simulink model "QuadSimUnity"  (R2015b)
settings: Solver=ode4  StartTime=0.0  StopTime=inf  FixedStep=Ts  RelTol=1e-3
values from neighbouring files (symbols this model uses):
  alpha1 = 10    [QuadSimInit.m]
  alpha2 = .5    (= 0.5)    [QuadSimInit.m]
  alpha3 = 10    [QuadSimInit.m]
  alpha4 = 0.5    [QuadSimInit.m]
  alpha5 = 10    [QuadSimInit.m]
  alpha6 = 0.5    [QuadSimInit.m]
  Am = -20*diag([1, 1, 1])    [QuadSimInit.m]
  b = 3.13e-5/2    (= 1.565e-05)    [QuadSimInit.m]
  Bm = inv(I)    [QuadSimInit.m]
  d = 7.5e-7/2    (= 3.75e-07)    [QuadSimInit.m]
  D_angle = 0.2    [QuadSimInit.m]
  Delay_Act = 0.003    [QuadSimInit.m]
  g = 9.81    [QuadSimInit.m]
  I_angle = 0.1    [QuadSimInit.m]
  Inverse_Psi_nom = Psi_nom.'*inv(Psi_nom*Psi_nom.')    [QuadSimInit.m]
  Ix_0 = 7.5e-3*1    (= 0.0075)    [QuadSimInit.m]
  Iy_0 = 6.5e-3*1    (= 0.0065)    [QuadSimInit.m]
  Iz_0 = 1.3e-2*1    (= 0.013)    [QuadSimInit.m]
  Jr = 6e-5    (= 6e-05)    [QuadSimInit.m]
  K = 100    [QuadSimInit.m]
  l = 0.23    [QuadSimInit.m]
  m = 0.650*4    (= 2.6)    [QuadSimInit.m]
  P_angle = 5    [QuadSimInit.m]
  Ts = 0.001    [QuadSimInit.m]
undefined symbols (not defined in the file or in its folder): a
libraries: simulink x9, etargetslib x5, dspnetwork x5, cstblocks x1, aerolibanimutils x1
settings Model: Creator=hyoon33  LastModifiedBy=lakshma2
settings SolverCC: AutoInsertRateTranBlk=on
settings DataIOCC: SaveFormat=Array
settings DebuggingCC: UnderspecifiedInitializationDetection=Classic  MergeDetectMultiDrivingBlocksExec=none  SolverPrmCheckMsg=warning  StateNameClashWarn=warning
settings HardwareCC: ProdBitPerPointer=32  ProdLargestAtomicFloat=None  ProdIntDivRoundTo=Undefined  ProdEndianess=Unspecified  ProdWordSize=32  ProdHWDeviceType=32-bit Generic
settings GRTTargetCC: GeneratePreprocessorConditionals=Disable all
settings ConfigComp: CovModelRefEnable=Off  CovSFcnEnable=off

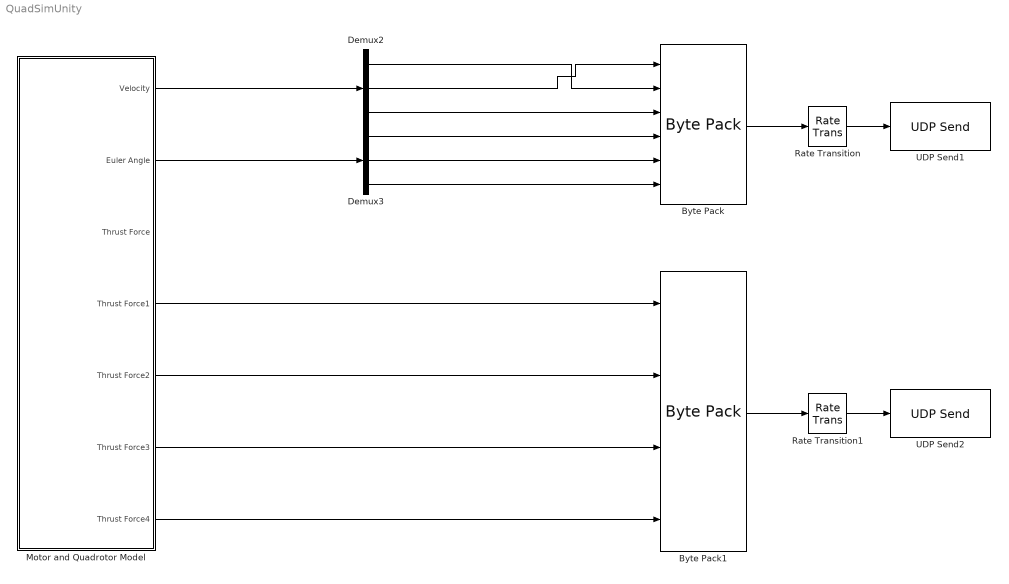
== system QuadSimUnity ==
  Byte Pack : etargetslib/Byte Pack  datatypes={'double','double','double','double','double','double'}  byteAlign=1
  Byte Pack1 : etargetslib/Byte Pack  datatypes={'double','double','double','double'}  byteAlign=1
  Demux2 : Demux  Outputs=3
  Demux3 : Demux  Outputs=3
  Motor and Quadrotor Model : Subsystem
  Rate Transition : RateTransition  OutPortSampleTime=0.016/16
  Rate Transition1 : RateTransition  OutPortSampleTime=0.016/16
  UDP Send1 : dspnetwork/UDP Send  remoteURL='127.0.0.1'  remotePort=25001  localURL='0.0.0.0'  localPortSource=Automatically determine  localPort=-1  sampletime=-1  separateLengthPort=0
  UDP Send2 : dspnetwork/UDP Send  remoteURL='127.0.0.1'  remotePort=25004  localURL='0.0.0.0'  localPortSource=Automatically determine  localPort=-1  sampletime=-1  separateLengthPort=0
  wires:
  Motor and Quadrotor Model/1(Velocity) -> Demux2/1
  Demux2/1 -> Byte Pack/2
  Demux3/2 -> Byte Pack/5
  Demux2/2 -> Byte Pack/1
  Demux3/1 -> Byte Pack/4
  Demux2/3 -> Byte Pack/3
  Demux3/3 -> Byte Pack/6
  Motor and Quadrotor Model/2(Euler Angle) -> Demux3/1
  Byte Pack/1 -> Rate Transition/1
  Rate Transition/1 -> UDP Send1/1
  Byte Pack1/1 -> Rate Transition1/1
  Rate Transition1/1 -> UDP Send2/1
  Motor and Quadrotor Model/4(Thrust Force1) -> Byte Pack1/1
  Motor and Quadrotor Model/5(Thrust Force2) -> Byte Pack1/2
  Motor and Quadrotor Model/6(Thrust Force3) -> Byte Pack1/3
  Motor and Quadrotor Model/7(Thrust Force4) -> Byte Pack1/4

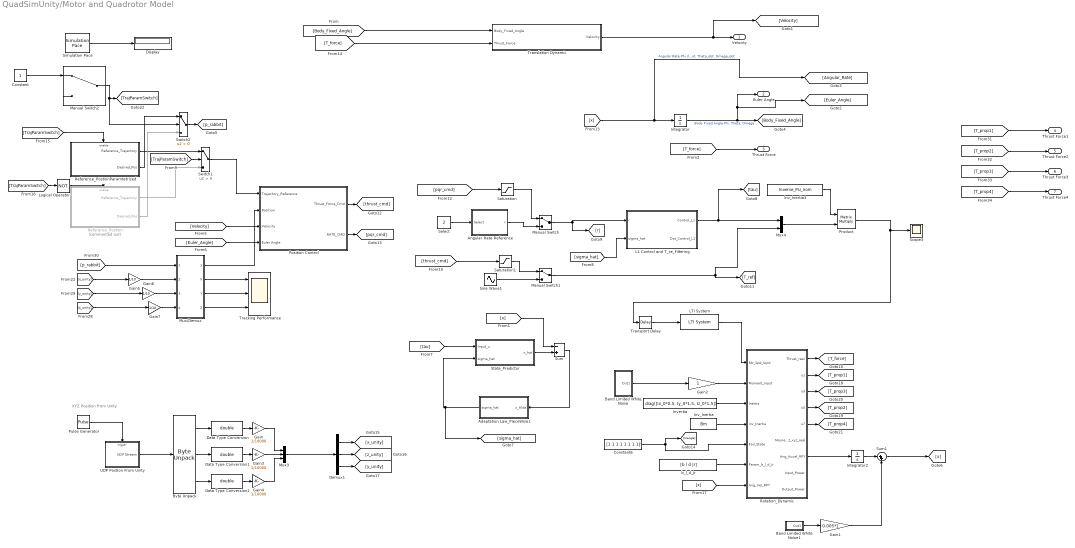
== system QuadSimUnity/Motor and Quadrotor Model ==
  note: XYZ Position from Unity
  Adaptation Law_PieceWise1 : Subsystem
  Angular Rate Reference : Subsystem
  Band Limited White Noise : Subsystem
  Band Limited White Noise1 : Subsystem
  Byte Unpack : etargetslib/Byte Unpack  dimensions={1,1,1}  datatypes={'int32','int32','int32'}  byteAlign=1
  Constant : Constant
  Constant6 : Constant  Value=[1 1 1 1 1 1 1 1]'
  Data Type Conversion : DataTypeConversion  OutDataTypeStr=double
  Data Type Conversion1 : DataTypeConversion  OutDataTypeStr=double
  Data Type Conversion2 : DataTypeConversion  OutDataTypeStr=double
  Demux1 : Demux  Outputs=3
  Display : Display
  Gain : Gain  Gain=1/10000
  Gain1 : Gain  Gain=0.005*1
  Gain2 : Gain
  Gain3 : Gain  Gain=1/10000
  Gain4 : Gain  Gain=1/10000
  Gain5 : Gain  Gain=1/10
  Gain6 : Gain  Gain=1/10
  Gain7 : Gain  Gain=1/10
  Integrator : Integrator
  Integrator2 : Integrator  InitialCondition=[0 0 0]'
  Inv_Inertia : Constant  Value=Bm  VectorParams1D=off
  Inv_Inertia3 : Constant  Value=Inverse_Psi_nom  VectorParams1D=off
  Invertia : Constant  Value=diag([Ix_0*0.5, Iy_0*1.5, Iz_0*1.5])  VectorParams1D=off
  L1 Control and T_re_Filtering : Subsystem
  LTI System : cstblocks/LTI System  sys=H_motor  IC=[]
  Logical Operator : Logic  Operator=NOT  AllPortsSameDT=off  OutDataTypeStr=boolean
  Manual Switch : ManualSwitch
  Manual Switch1 : ManualSwitch
  Manual Switch2 : ManualSwitch
  Mux/Demux : Subsystem
  Mux3 : Mux  Inputs=3
  Mux4 : Mux  Inputs=2
  Position Control : Subsystem
  Product : Product  Multiplication=Matrix(*)
  Pulse Generator : DiscretePulseGenerator  PulseType=Time based  Period=1/50  PulseWidth=50
  Reference_Postion : Subsystem  Commented=on
  Reference_PostionParamtetrized : Subsystem
  Rotation_Dynamic : MATLAB Function  TreatAsAtomicUnit=on
  Saturation : Saturate  UpperLimit=10  LowerLimit=-10
  Saturation1 : Saturate  UpperLimit=100  LowerLimit=-100
  Scope3 : Scope
  Select : Constant  Value=2
  Simulation Pace : aerolibanimutils/Simulation Pace  SimulationPace=1  SleepMode=MATLAB Thread  OutputPaceError=on  SampleTime=-1
      settings: AttributesFormatString=%<SimulationPace> sec/sec
  Sine Wave1 : Sin  Amplitude=0  Bias=m*9.81  Frequency=2  SampleTime=0
  State_Predictor : Subsystem
  Sum : Sum  Inputs=-+
  Sum1 : Sum  Inputs=|++
  Switch1 : Switch  Criteria=u2 > Threshold
  Switch2 : Switch  Criteria=u2 > Threshold
  Tracking Performance : Scope  NumInputPorts=3
  Translation Dynamic : Subsystem
  Transport Delay : TransportDelay  DelayTime=Delay_Act
  UDP Postion From Unity : Subsystem
  b_l_d_Jr : Constant  Value=[b l d Jr]
  Velocity : Outport
  Euler Angle : Outport  Port=2
  Thrust Force : Outport  Port=3
  Thrust Force1 : Outport  Port=4
  Thrust Force2 : Outport  Port=5
  Thrust Force3 : Outport  Port=6
  Thrust Force4 : Outport  Port=7
  wires:
  [Velocity] -> Position Control/3(Velocity)
  [Euler_Angle] -> Position Control/4(Euler Angle)
  [x] -> Integrator/1, [Angular_Rate]  "Angular Rate Phi dot, Theta_dot, Omega_dot"
  Integrator/1 -> Euler Angle/1, [Euler_Angle], [Body_Fixed_Angle]  "Body Fixed Angle Phi, Theta, Omega"
  [Body_Fixed_Angle] -> Translation Dynamic/1(Body_Fixed_Angle)
  b_l_d_Jr/1 -> Rotation_Dynamic/6(Param_b_l_d_Jr)
  Invertia/1 -> Rotation_Dynamic/3(Inertia)
  Inv_Inertia/1 -> Rotation_Dynamic/4(inv_Inertia)
  Rotation_Dynamic/7(Ang_Accel_RPY) -> Integrator2/1
  Manual Switch/1 -> L1 Control and T_re_Filtering/1(r), [r]
  Select/1 -> Angular Rate Reference/1(Select)
  [sigma_hat] -> L1 Control and T_re_Filtering/2(sigma_hat)
  L1 Control and T_re_Filtering/1(Control_L1) -> Mux4/1, [tau]
  Integrator2/1 -> Sum1/1
  Band Limited White Noise/1(Out1) -> Gain2/1
  Gain2/1 -> Rotation_Dynamic/2(Moment_Input)
  Transport Delay/1 -> LTI System/1
  LTI System/1 -> Rotation_Dynamic/1(Rtr_Spd_Sqrd)
  Constant6/1 -> [triangle], Rotation_Dynamic/5(Fail_State)
  State_Predictor/1(x_hat) -> Sum/2
  [x] -> Sum/1
  Sum/1 -> Adaptation Law_PieceWise1/1(x_tilda)
  Adaptation Law_PieceWise1/1(sigma_hat) -> [sigma_hat], State_Predictor/2(sigma_hat)
  Rotation_Dynamic/1(Thrust_real) -> [T_force]
  [tau] -> State_Predictor/1(input_u)
  Manual Switch1/1 -> Mux4/2, [T_ref]
  Angular Rate Reference/1(r) -> Manual Switch/2
  [pqr_cmd] -> Saturation/1
  Sine Wave1/1 -> Manual Switch1/2
  [thrust_cmd] -> Saturation1/1
  Saturation/1 -> Manual Switch/1
  Saturation1/1 -> Manual Switch1/1
  Position Control/1(Thrust_Force_Cmd) -> [thrust_cmd]
  Position Control/2(RATE_CMD) -> [pqr_cmd]
  [T_force] -> Translation Dynamic/2(Thrust_Force)
  Sum1/1 -> [x]
  Band Limited White Noise1/1(Out1) -> Gain1/1
  Gain1/1 -> Sum1/2
  Translation Dynamic/1(Velocity) -> [Velocity], Velocity/1
  Product/1 -> Transport Delay/1, Scope3/1
  [x] -> Rotation_Dynamic/7(Ang_Vel_RPY)
  Mux4/1 -> Product/2
  Inv_Inertia3/1 -> Product/1
  Byte Unpack/1 -> Data Type Conversion/1
  Byte Unpack/2 -> Data Type Conversion1/1
  Byte Unpack/3 -> Data Type Conversion2/1
  Simulation Pace/1 -> Display/1
  UDP Postion From Unity/1(UDP Stream) -> Byte Unpack/1
  Pulse Generator/1 -> UDP Postion From Unity/Trigger
  Gain/1 -> Mux3/1
  Gain3/1 -> Mux3/2
  Gain4/1 -> Mux3/3
  Data Type Conversion/1 -> Gain/1
  Data Type Conversion1/1 -> Gain3/1
  Data Type Conversion2/1 -> Gain4/1
  [p_rabbit] -> Mux/Demux/1(Rabbit)
  [x_unity] -> Gain5/1
  [y_unity] -> Gain6/1
  [z_unity] -> Gain7/1
  Mux/Demux/1(Position) -> Position Control/2(Position)
  Mux/Demux/2(X) -> Tracking Performance/1
  Mux/Demux/3(Y) -> Tracking Performance/2
  Mux/Demux/4(Z) -> Tracking Performance/3
  [T_force] -> Thrust Force/1
  Gain5/1 -> Mux/Demux/2(XUnity)
  Gain6/1 -> Mux/Demux/3(YUnity)
  Gain7/1 -> Mux/Demux/4(ZUnity)
  Mux3/1 -> Demux1/1
  Demux1/1 -> [x_unity]
  Demux1/2 -> [z_unity]
  Demux1/3 -> [y_unity]
  Rotation_Dynamic/2(u1) -> [T_prop1]
  Rotation_Dynamic/4(u5) -> [T_prop2]
  Rotation_Dynamic/3(u3) -> [T_prop3]
  Rotation_Dynamic/5(u7) -> [T_prop4]
  [T_prop1] -> Thrust Force1/1
  [T_prop2] -> Thrust Force2/1
  [T_prop3] -> Thrust Force3/1
  [T_prop4] -> Thrust Force4/1
  Switch1/1 -> Position Control/1(Trajectory_Reference)
  Reference_Postion/1(Reference_Trajectory) -> Switch1/3
  Reference_PostionParamtetrized/1(Reference_Trajectory) -> Switch1/1
  Reference_PostionParamtetrized/2(Desired_Pos) -> Switch2/1
  Reference_Postion/2(Desired_Pos) -> Switch2/3
  Switch2/1 -> [p_rabbit]
  Manual Switch2/1 -> Switch2/2, [TrajParamSwitch]
  Constant/1 -> Manual Switch2/1
  [TrajParamSwitch] -> Switch1/2
  [TrajParamSwitch] -> Reference_PostionParamtetrized/Enable
  [TrajParamSwitch] -> Logical Operator/1
  Logical Operator/1 -> Reference_Postion/Enable

== system QuadSimUnity/Motor and Quadrotor Model/Adaptation Law_PieceWise1 ==
  x_tilda : Inport
  -inv(Bm)*inv(Phi_Ts)*exp_Am_Ts : Constant  Value=inv(Bm)*inv(inv(Am)*(expm(Am*Ts)-eye(3)))*(expm(Am*Ts))
  Gain3 : Gain  Gain=-1
  Product6 : Product  Multiplication=Matrix(*)
  Rate Transition : RateTransition  OutPortSampleTime=Ts
  Rate Transition1 : RateTransition  OutPortSampleTimeOpt=Inherit  OutPortSampleTime=Ts
  Rate Transition3 : RateTransition  X0=inv(Bm)*inv(inv(Am)*(exp(Am*Ts)-eye(3)))*(exp(Am*Ts))  OutPortSampleTime=Ts
  Saturation2 : Saturate  Commented=through  UpperLimit=10000  LowerLimit=-10000
  sigma_hat : Outport
  wires:
  Saturation2/1 -> sigma_hat/1
  Rate Transition3/1 -> Product6/1
  Gain3/1 -> Rate Transition1/1
  Rate Transition1/1 -> Saturation2/1
  -inv(Bm)*inv(Phi_Ts)*exp_Am_Ts/1 -> Rate Transition3/1
  x_tilda/1 -> Rate Transition/1
  Product6/1 -> Gain3/1
  Rate Transition/1 -> Product6/2

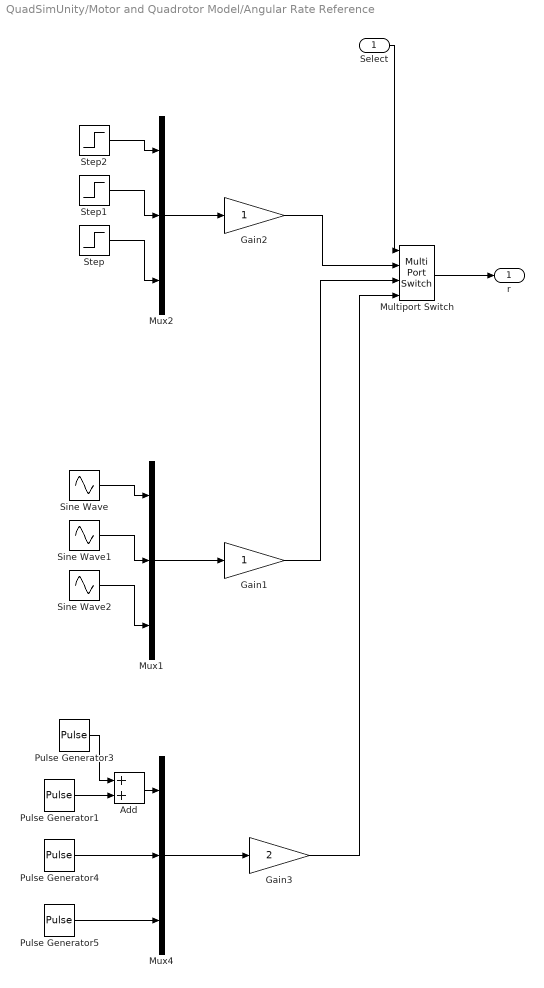
== system QuadSimUnity/Motor and Quadrotor Model/Angular Rate Reference ==
  Select : Inport
  Add : Sum
  Gain1 : Gain
  Gain2 : Gain
  Gain3 : Gain  Gain=2
  Multiport Switch : MultiPortSwitch
  Mux1 : Mux  Inputs=3
  Mux2 : Mux  Inputs=3
  Mux4 : Mux  Inputs=3
  Pulse Generator1 : DiscretePulseGenerator  PulseType=Time based  Amplitude=-1  Period=10  PhaseDelay=10
  Pulse Generator3 : DiscretePulseGenerator  PulseType=Time based  Period=10  PhaseDelay=1
  Pulse Generator4 : DiscretePulseGenerator  PulseType=Time based  Amplitude=0  Period=6  PulseWidth=40  PhaseDelay=1.5
  Pulse Generator5 : DiscretePulseGenerator  PulseType=Time based  Amplitude=0  Period=7  PulseWidth=40  PhaseDelay=2
  Sine Wave : Sin  Frequency=2  SampleTime=0
  Sine Wave1 : Sin  Frequency=2  Phase=pi  SampleTime=0
  Sine Wave2 : Sin  Amplitude=0  Frequency=2  SampleTime=0
  Step : Step  Time=3  After=0  SampleTime=0
  Step1 : Step  Time=2  SampleTime=0
  Step2 : Step  SampleTime=0
  r : Outport
  wires:
  Sine Wave/1 -> Mux1/1
  Sine Wave1/1 -> Mux1/2
  Sine Wave2/1 -> Mux1/3
  Step2/1 -> Mux2/1
  Step1/1 -> Mux2/2
  Step/1 -> Mux2/3
  Mux1/1 -> Gain1/1
  Mux2/1 -> Gain2/1
  Select/1 -> Multiport Switch/1
  Gain2/1 -> Multiport Switch/2
  Pulse Generator4/1 -> Mux4/2
  Pulse Generator5/1 -> Mux4/3
  Mux4/1 -> Gain3/1
  Gain1/1 -> Multiport Switch/3
  Gain3/1 -> Multiport Switch/4
  Multiport Switch/1 -> r/1
  Add/1 -> Mux4/1
  Pulse Generator3/1 -> Add/1
  Pulse Generator1/1 -> Add/2

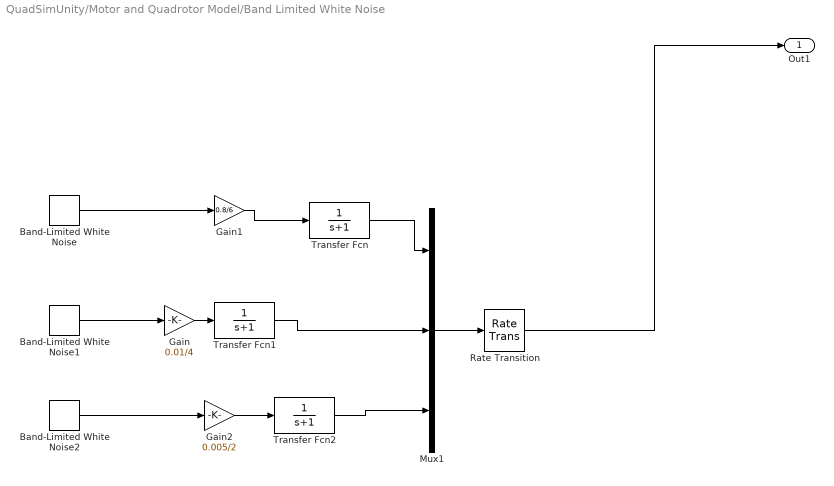
== system QuadSimUnity/Motor and Quadrotor Model/Band Limited White Noise ==
  Band-Limited White Noise : simulink/Sources/Band-Limited White Noise  Cov=[.1]  Ts=Ts  seed=[23341]
  Band-Limited White Noise1 : simulink/Sources/Band-Limited White Noise  Cov=[.1]  Ts=Ts  seed=[24451]
  Band-Limited White Noise2 : simulink/Sources/Band-Limited White Noise  Cov=[.1]  Ts=Ts  seed=[87745]
  Gain : Gain  Gain=0.01/4
  Gain1 : Gain  Gain=0.8/6
  Gain2 : Gain  Gain=0.005/2
  Mux1 : Mux  Inputs=3
  Rate Transition : RateTransition
  Transfer Fcn : TransferFcn  Denominator=[1 1]
  Transfer Fcn1 : TransferFcn  Denominator=[1 1]
  Transfer Fcn2 : TransferFcn  Denominator=[1 1]
  Out1 : Outport
  wires:
  Rate Transition/1 -> Out1/1
  Band-Limited White Noise/1 -> Gain1/1
  Band-Limited White Noise1/1 -> Gain/1
  Band-Limited White Noise2/1 -> Gain2/1
  Mux1/1 -> Rate Transition/1
  Gain/1 -> Transfer Fcn1/1
  Gain1/1 -> Transfer Fcn/1
  Gain2/1 -> Transfer Fcn2/1
  Transfer Fcn/1 -> Mux1/1
  Transfer Fcn1/1 -> Mux1/2
  Transfer Fcn2/1 -> Mux1/3

== system QuadSimUnity/Motor and Quadrotor Model/Band Limited White Noise1 ==
  Band-Limited White Noise : simulink/Sources/Band-Limited White Noise  Cov=[0.1]  Ts=0.1  seed=[23341]
  Band-Limited White Noise1 : simulink/Sources/Band-Limited White Noise  Cov=[0.1]  Ts=0.1  seed=[23241]
  Band-Limited White Noise2 : simulink/Sources/Band-Limited White Noise  Cov=[0.1]  Ts=0.1  seed=[21341]
  Mux : Mux  Inputs=3
  Rate Transition : RateTransition
  Out1 : Outport
  wires:
  Rate Transition/1 -> Out1/1
  Band-Limited White Noise1/1 -> Mux/3
  Band-Limited White Noise/1 -> Mux/1
  Mux/1 -> Rate Transition/1
  Band-Limited White Noise2/1 -> Mux/2

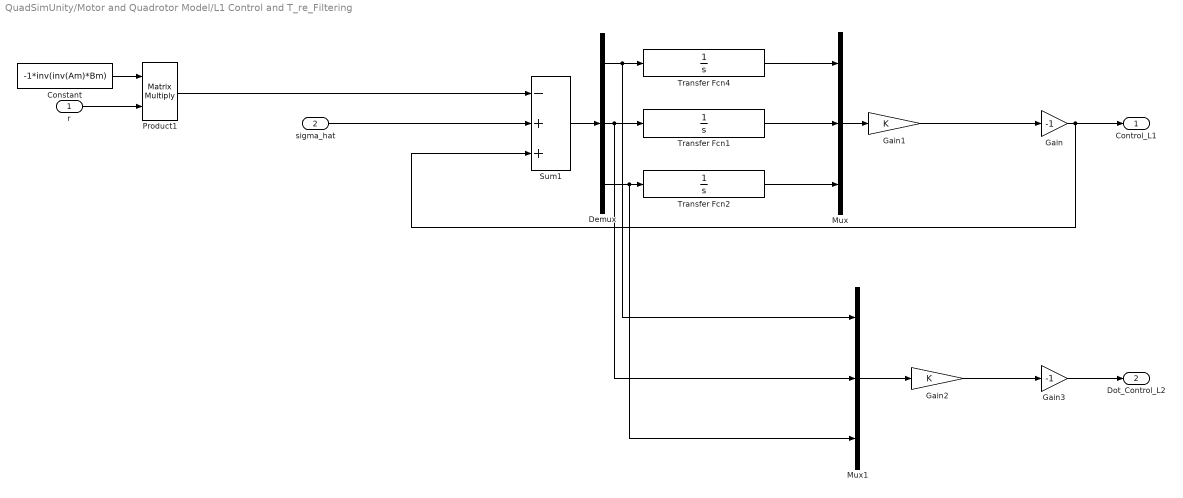
== system QuadSimUnity/Motor and Quadrotor Model/L1 Control and T_re_Filtering ==
  r : Inport
  sigma_hat : Inport  Port=2
  Constant : Constant  Value=-1*inv(inv(Am)*Bm)
  Demux : Demux  Outputs=3
  Gain : Gain  Gain=-1
  Gain1 : Gain  Gain=K
  Gain2 : Gain  Gain=K
  Gain3 : Gain  Gain=-1
  Mux : Mux  Inputs=3
  Mux1 : Mux  Inputs=3
  Product1 : Product  Multiplication=Matrix(*)
  Sum1 : Sum  Inputs=-++
  Transfer Fcn1 : TransferFcn  Denominator=[1 0]
  Transfer Fcn2 : TransferFcn  Denominator=[1 0]
  Transfer Fcn4 : TransferFcn  Denominator=[1 0]
  Control_L1 : Outport
  Dot_Control_L2 : Outport  Port=2
  wires:
  r/1 -> Product1/2
  Sum1/1 -> Demux/1
  Demux/1 -> Mux1/1, Transfer Fcn4/1
  Demux/2 -> Mux1/2, Transfer Fcn1/1
  Demux/3 -> Mux1/3, Transfer Fcn2/1
  Mux/1 -> Gain1/1
  Transfer Fcn4/1 -> Mux/1
  Transfer Fcn1/1 -> Mux/2
  Transfer Fcn2/1 -> Mux/3
  Constant/1 -> Product1/1
  sigma_hat/1 -> Sum1/2
  Gain/1 -> Sum1/3, Control_L1/1
  Product1/1 -> Sum1/1
  Gain1/1 -> Gain/1
  Mux1/1 -> Gain2/1
  Gain2/1 -> Gain3/1
  Gain3/1 -> Dot_Control_L2/1

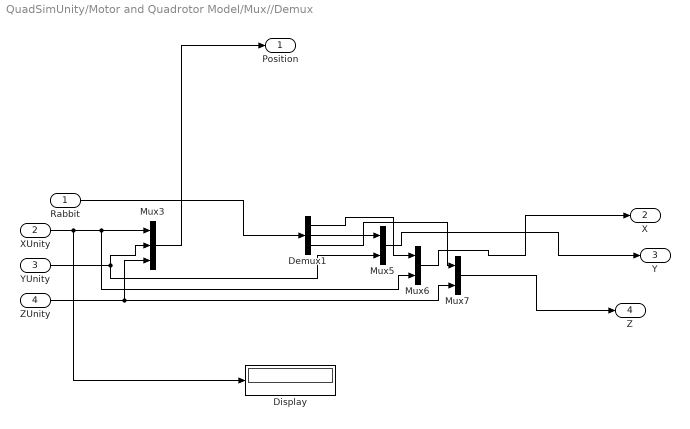
== system QuadSimUnity/Motor and Quadrotor Model/Mux//Demux ==
  Rabbit : Inport
  XUnity : Inport  Port=2
  YUnity : Inport  Port=3
  ZUnity : Inport  Port=4
  Demux1 : Demux  Outputs=3
  Display : Display
  Mux3 : Mux  Inputs=3
  Mux5 : Mux  Inputs=2
  Mux6 : Mux  Inputs=2
  Mux7 : Mux  Inputs=2
  Position : Outport
  X : Outport  Port=2
  Y : Outport  Port=3
  Z : Outport  Port=4
  wires:
  Demux1/1 -> Mux6/1
  Mux7/1 -> Z/1
  Mux6/1 -> X/1
  Demux1/2 -> Mux5/1
  Mux3/1 -> Position/1
  ZUnity/1 -> Mux3/3, Mux7/2
  YUnity/1 -> Mux3/2, Mux5/2
  XUnity/1 -> Display/1, Mux6/2, Mux3/1
  Demux1/3 -> Mux7/1
  Mux5/1 -> Y/1
  Rabbit/1 -> Demux1/1

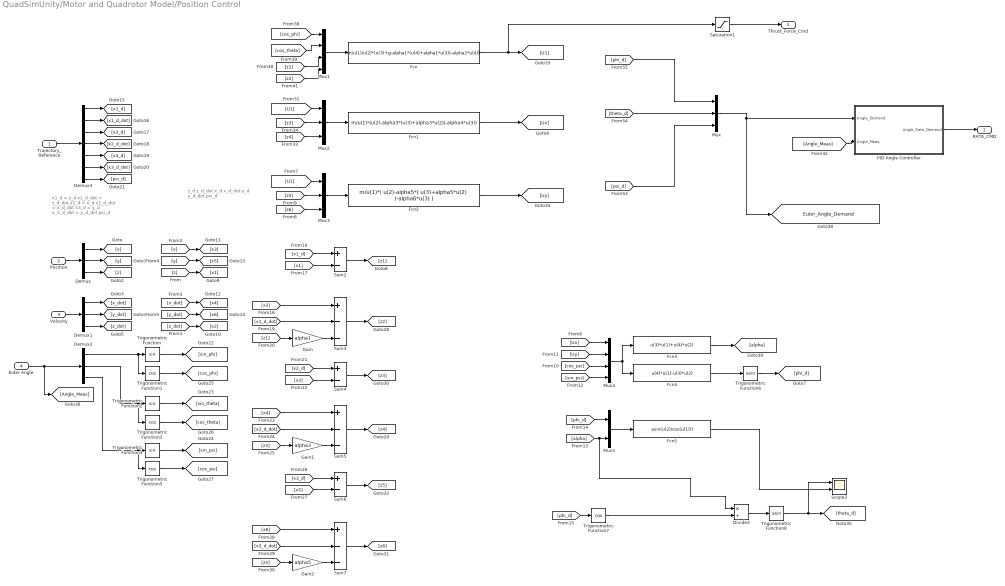
== system QuadSimUnity/Motor and Quadrotor Model/Position Control ==
  note: x1_d =  z_d
      | x1_d_dot = z_d_dot
      |
      | x2_d = x_d
      | x2_d_dot = x_d_dot
      |
      | x3_d = y_d
      | x_3_d_dot = y_d_dot
      |
      | psi_d
  note: z_d
      | z_d_dot
      |
      | x_d
      | x_d_dot
      |
      | y_d
      | y_d_dot
      |
      | psi_d
  Trajectory_Reference : Inport
  Position : Inport  Port=2
  Velocity : Inport  Port=3
  Euler Angle : Inport  Port=4
  Demux : Demux  Outputs=3
  Demux1 : Demux  Outputs=3
  Demux2 : Demux  Outputs=3
  Demux3 : Demux  Outputs=7
  Divide3 : Product  Inputs=*/
  Fcn : Fcn  Expr=m/u(1)/u(2)*(u(3)+g-alpha1*(u(4)+alpha1*u(3))-alpha2*u(4))
  Fcn1 : Fcn  Expr=m/u(1)*(u(2)-alpha3*(u(3)+alpha3*u(2))-alpha4*u(3))
  Fcn2 : Fcn  Expr=m/u(1)*( u(2)-alpha5*( u(3)+alpha5*u(2) )-alpha6*u(3) )
  Fcn3 : Fcn  Expr=u(3)*u(1)+u(4)*u(2)
  Fcn4 : Fcn  Expr=u(4)*u(1)-u(3)*u(2)
  Fcn5 : Fcn  Expr=asin(u(2)/cos(u(1)))
  Gain : Gain  Gain=alpha1
  Gain1 : Gain  Gain=alpha3
  Gain2 : Gain  Gain=alpha5
  Mux : Mux  Inputs=3
  Mux1 : Mux
  Mux2 : Mux  Inputs=3
  Mux3 : Mux  Inputs=3
  Mux4 : Mux
  Mux5 : Mux  Inputs=2
  PID Angle Controller : Subsystem
  Saturation1 : Saturate  UpperLimit=30  LowerLimit=-30
  Scope3 : Scope  NumInputPorts=2
  Sum2 : Sum  Inputs=+-
  Sum3 : Sum  Inputs=+--
  Sum4 : Sum  Inputs=+-
  Sum5 : Sum  Inputs=+--
  Sum6 : Sum  Inputs=+-
  Sum7 : Sum  Inputs=+--
  Trigonometric Function : Trigonometry
  Trigonometric Function{1,3,5,7} (4 alike) : Trigonometry  Operator=cos
  Trigonometric Function2 : Trigonometry
  Trigonometric Function4 : Trigonometry
  Trigonometric Function6 : Trigonometry  Operator=asin
  Trigonometric Function8 : Trigonometry  Operator=asin
  Thrust_Force_Cmd : Outport
  RATE_CMD : Outport  Port=2
  tag scope: Euler_Angle_Demand=global
  wires:
  Position/1 -> Demux/1
  Velocity/1 -> Demux1/1
  Euler Angle/1 -> [Angle_Meas], Demux2/1
  Demux/1 -> [x]
  Demux/2 -> [y]
  Demux/3 -> [z]
  Demux1/1 -> [x_dot]
  Demux1/2 -> [y_dot]
  Demux1/3 -> [z_dot]
  [z] -> [x1]
  [z_dot] -> [x2]
  [x] -> [x3]
  [x_dot] -> [x4]
  [y] -> [x5]
  [y_dot] -> [x6]
  Trajectory_Reference/1 -> Demux3/1
  Demux3/1 -> [x1_d]
  Demux3/2 -> [x1_d_dot]
  Demux3/3 -> [x2_d]
  Demux3/4 -> [x2_d_dot]
  Demux3/5 -> [x3_d]
  Demux3/6 -> [x3_d_dot]
  Demux3/7 -> [psi_d]
  Demux2/1 -> Trigonometric Function1/1, Trigonometric Function/1
  Trigonometric Function/1 -> [sin_phi]
  Trigonometric Function1/1 -> [cos_phi]
  Demux2/2 -> Trigonometric Function3/1, Trigonometric Function2/1
  Trigonometric Function2/1 -> [sin_theta]
  Trigonometric Function3/1 -> [cos_theta]
  Trigonometric Function4/1 -> [sin_psi]
  Trigonometric Function5/1 -> [cos_psi]
  Demux2/3 -> Trigonometric Function5/1, Trigonometric Function4/1
  [x1_d] -> Sum2/1
  [x1] -> Sum2/2
  Sum2/1 -> [z1]
  [x1_d_dot] -> Sum3/2
  [x2] -> Sum3/1
  Gain/1 -> Sum3/3
  [z1] -> Gain/1
  Sum3/1 -> [z2]
  [x2_d] -> Sum4/1
  [x3] -> Sum4/2
  Sum4/1 -> [z3]
  [x2_d_dot] -> Sum5/2
  [x4] -> Sum5/1
  Gain1/1 -> Sum5/3
  [z3] -> Gain1/1
  Sum5/1 -> [z4]
  [x3_d] -> Sum6/1
  [x5] -> Sum6/2
  Sum6/1 -> [z5]
  [x3_d_dot] -> Sum7/2
  [x6] -> Sum7/1
  Gain2/1 -> Sum7/3
  [z5] -> Gain2/1
  Sum7/1 -> [z6]
  [alpha] -> Divide3/1, Mux5/2
  Trigonometric Function7/1 -> Divide3/2
  Divide3/1 -> Trigonometric Function8/1
  Trigonometric Function8/1 -> Scope3/1, [theta_d]
  Mux1/1 -> Fcn/1
  [cos_phi] -> Mux1/1
  [cos_theta] -> Mux1/2
  [z1] -> Mux1/3
  [z2] -> Mux1/4
  Mux2/1 -> Fcn1/1
  [U1] -> Mux2/1
  [z4] -> Mux2/3
  [z3] -> Mux2/2
  Fcn1/1 -> [Ux]
  Mux3/1 -> Fcn2/1
  [U1] -> Mux3/1
  [z6] -> Mux3/3
  [z5] -> Mux3/2
  Fcn2/1 -> [Uy]
  Mux4/1 -> Fcn4/1, Fcn3/1
  [Ux] -> Mux4/1
  [cos_psi] -> Mux4/3
  [Uy] -> Mux4/2
  [sin_psi] -> Mux4/4
  Fcn4/1 -> Trigonometric Function6/1
  Trigonometric Function6/1 -> [phi_d]
  Fcn3/1 -> [alpha]
  [phi_d] -> Mux5/1
  Mux5/1 -> Fcn5/1
  Fcn5/1 -> Scope3/2
  [phi_d] -> Trigonometric Function7/1
  [phi_d] -> Mux/1
  [theta_d] -> Mux/2
  [psi_d] -> Mux/3
  Mux/1 -> PID Angle Controller/1(Angle_Demand), [Euler_Angle_Demand]
  [Angle_Meas] -> PID Angle Controller/2(Angle_Meas.)
  Saturation1/1 -> Thrust_Force_Cmd/1
  Fcn/1 -> Saturation1/1, [U1]
  PID Angle Controller/1(Angle_Rate_Demand) -> RATE_CMD/1

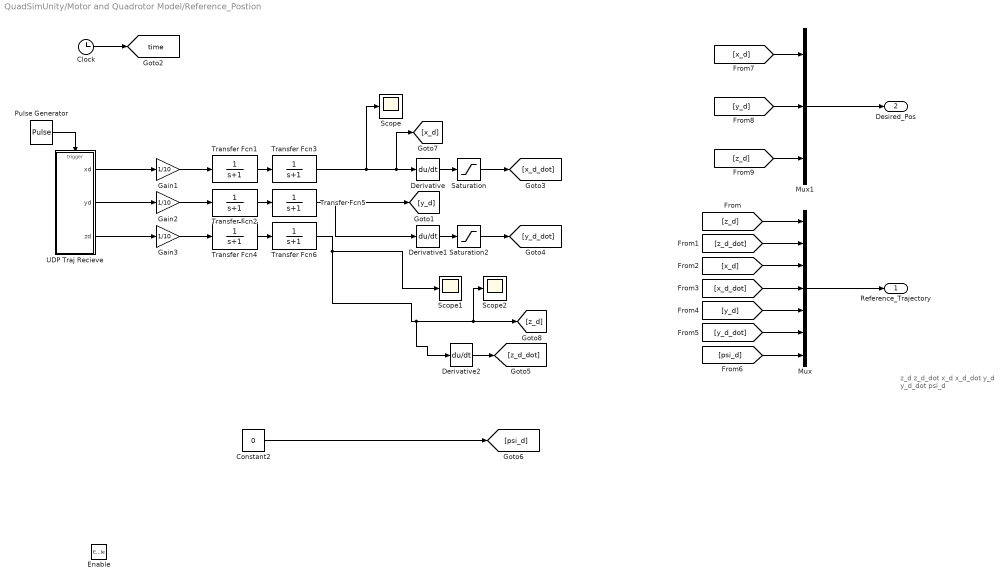
== system QuadSimUnity/Motor and Quadrotor Model/Reference_Postion ==
  note: z_d
      | z_d_dot
      |
      | x_d
      | x_d_dot
      |
      | y_d
      | y_d_dot
      |
      | psi_d
  Enable : EnablePort
  Clock : Clock
  Constant2 : Constant  Value=0
  Derivative : Derivative  CoefficientInTFapproximation=300
  Derivative1 : Derivative  CoefficientInTFapproximation=500
  Derivative2 : Derivative  CoefficientInTFapproximation=500
  Gain1 : Gain  Gain=1/10
  Gain2 : Gain  Gain=1/10
  Gain3 : Gain  Gain=1/10
  Mux : Mux  Inputs=7
  Mux1 : Mux  Inputs=3
  Pulse Generator : DiscretePulseGenerator  PulseType=Time based  Period=1/10  PulseWidth=50
  Saturation : Saturate  UpperLimit=5  LowerLimit=-5
  Saturation2 : Saturate  UpperLimit=5  LowerLimit=-5
  Scope : Scope
  Scope1 : Scope
  Scope2 : Scope
  Transfer Fcn{1..6} (6 alike) : TransferFcn  Denominator=[1 1]
  UDP Traj Recieve : Subsystem
  Reference_Trajectory : Outport
  Desired_Pos : Outport  Port=2
  tag scope: time=global
  wires:
  Constant2/1 -> [psi_d]
  Mux/1 -> Reference_Trajectory/1
  [z_d] -> Mux/1
  [z_d_dot] -> Mux/2
  [x_d] -> Mux/3
  [x_d_dot] -> Mux/4
  [y_d] -> Mux/5
  [y_d_dot] -> Mux/6
  [psi_d] -> Mux/7
  Derivative/1 -> Saturation/1
  Derivative1/1 -> Saturation2/1
  [x_d] -> Mux1/1
  [y_d] -> Mux1/2
  [z_d] -> Mux1/3
  Mux1/1 -> Desired_Pos/1
  Clock/1 -> [time]
  Transfer Fcn4/1 -> Transfer Fcn6/1
  Transfer Fcn2/1 -> Transfer Fcn5/1
  Transfer Fcn1/1 -> Transfer Fcn3/1
  Pulse Generator/1 -> UDP Traj Recieve/Trigger
  Saturation/1 -> [x_d_dot]
  UDP Traj Recieve/1(xd) -> Gain1/1
  UDP Traj Recieve/2(yd) -> Gain2/1
  UDP Traj Recieve/3(zd) -> Gain3/1
  Derivative2/1 -> [z_d_dot]
  Gain1/1 -> Transfer Fcn1/1
  Gain2/1 -> Transfer Fcn2/1
  Gain3/1 -> Transfer Fcn4/1
  Saturation2/1 -> [y_d_dot]
  Transfer Fcn3/1 -> Scope/1, [x_d], Derivative/1
  Transfer Fcn5/1 -> [y_d], Derivative1/1
  Transfer Fcn6/1 -> Derivative2/1, Scope2/1, [z_d], Scope1/1

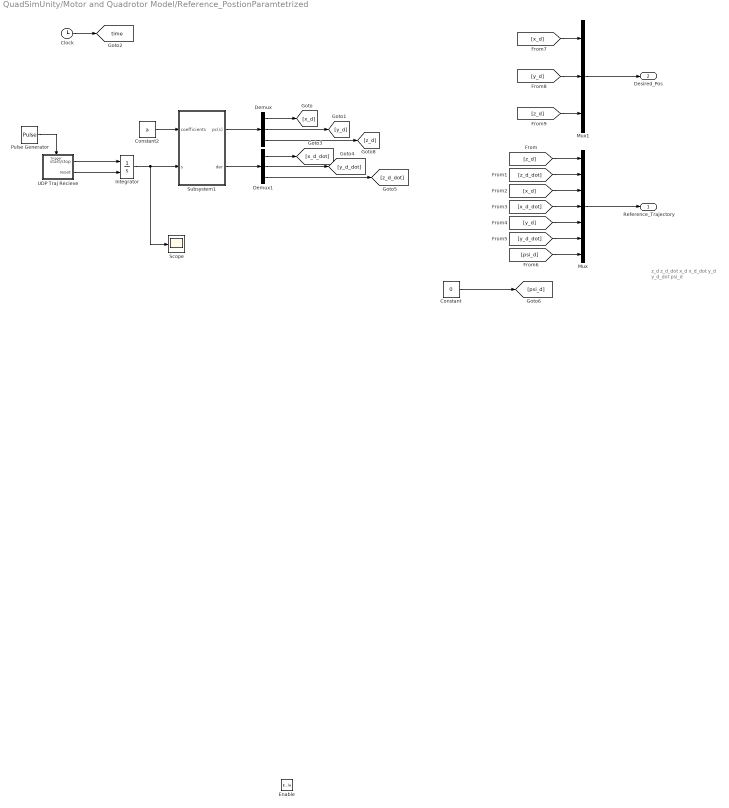
== system QuadSimUnity/Motor and Quadrotor Model/Reference_PostionParamtetrized ==
  note: z_d
      | z_d_dot
      |
      | x_d
      | x_d_dot
      |
      | y_d
      | y_d_dot
      |
      | psi_d
  Enable : EnablePort
  Clock : Clock
  Constant : Constant  Value=0
  Constant2 : Constant  Value=a
  Demux : Demux  Outputs=3
  Demux1 : Demux  Outputs=3
  Integrator : Integrator  ExternalReset=either
  Mux : Mux  Inputs=7
  Mux1 : Mux  Inputs=3
  Pulse Generator : DiscretePulseGenerator  PulseType=Time based  Period=1/50  PulseWidth=50
  Scope : Scope
  Subsystem1 : Subsystem
  UDP Traj Recieve : Subsystem
  Reference_Trajectory : Outport
  Desired_Pos : Outport  Port=2
  tag scope: time=global
  wires:
  Mux/1 -> Reference_Trajectory/1
  [z_d] -> Mux/1
  [z_d_dot] -> Mux/2
  [x_d] -> Mux/3
  [x_d_dot] -> Mux/4
  [y_d] -> Mux/5
  [y_d_dot] -> Mux/6
  [psi_d] -> Mux/7
  [x_d] -> Mux1/1
  [y_d] -> Mux1/2
  [z_d] -> Mux1/3
  Mux1/1 -> Desired_Pos/1
  Clock/1 -> [time]
  Pulse Generator/1 -> UDP Traj Recieve/Trigger
  Demux1/1 -> [x_d_dot]
  UDP Traj Recieve/1(start/stop) -> Integrator/1
  Demux1/2 -> [y_d_dot]
  Constant/1 -> [psi_d]
  Subsystem1/1(pc(s)) -> Demux/1
  Demux/1 -> [x_d]
  Demux/2 -> [y_d]
  Demux/3 -> [z_d]
  Subsystem1/2(der) -> Demux1/1
  Demux1/3 -> [z_d_dot]
  Constant2/1 -> Subsystem1/1(coefficients)
  UDP Traj Recieve/2(reset) -> Integrator/2
  Integrator/1 -> Scope/1, Subsystem1/2(s)

== system QuadSimUnity/Motor and Quadrotor Model/State_Predictor ==
  input_u : Inport
  sigma_hat : Inport  Port=2
  Am : Constant  Value=Am
  Constant4 : Constant  Value=Bm
  Integrator : Integrator
  Product : Product  Multiplication=Matrix(*)  RndMeth=Zero
  Product6 : Product  Multiplication=Matrix(*)
  Sum : Sum
  Sum1 : Sum
  x_hat : Outport
  wires:
  Product6/1 -> Sum/1
  Product/1 -> Sum/2
  Sum1/1 -> Product6/2
  Constant4/1 -> Product6/1
  Sum/1 -> Integrator/1
  input_u/1 -> Sum1/1
  Am/1 -> Product/1
  Integrator/1 -> x_hat/1, Product/2
  sigma_hat/1 -> Sum1/2

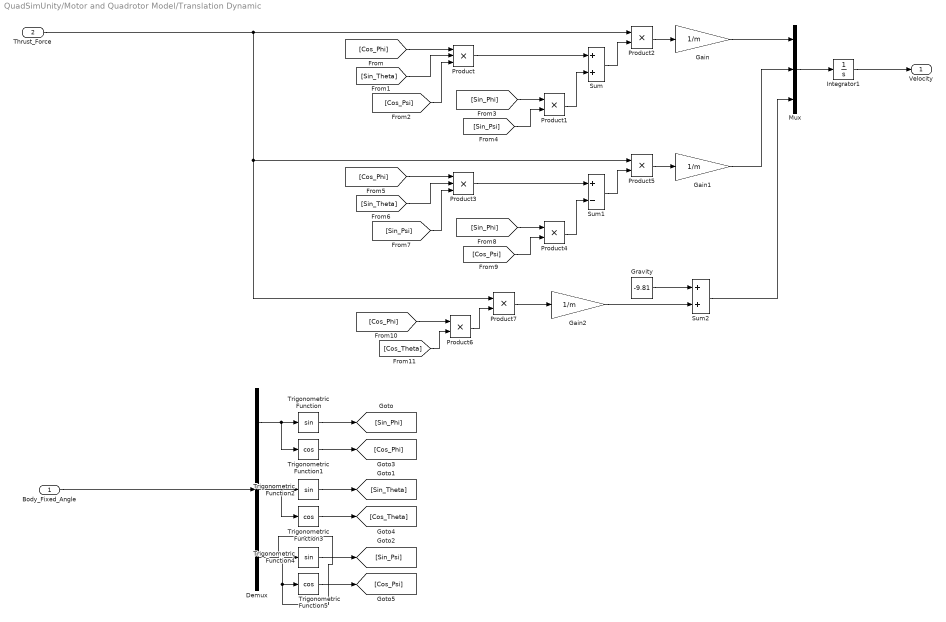
== system QuadSimUnity/Motor and Quadrotor Model/Translation Dynamic ==
  Body_Fixed_Angle : Inport
  Thrust_Force : Inport  Port=2
  Demux : Demux  Outputs=3
  Gain : Gain  Gain=1/m
  Gain1 : Gain  Gain=1/m
  Gain2 : Gain  Gain=1/m
  Gravity : Constant  Value=-9.81
  Integrator1 : Integrator  InitialCondition=[0 0 0]
  Mux : Mux  Inputs=3
  Product : Product  Inputs=3
  Product{1..2,4..7} (6 alike) : Product
  Product3 : Product  Inputs=3
  Sum : Sum
  Sum1 : Sum  Inputs=+-
  Sum2 : Sum
  Trigonometric Function : Trigonometry
  Trigonometric Function1 : Trigonometry  Operator=cos
  Trigonometric Function2 : Trigonometry
  Trigonometric Function3 : Trigonometry  Operator=cos
  Trigonometric Function4 : Trigonometry
  Trigonometric Function5 : Trigonometry  Operator=cos
  Velocity : Outport
  wires:
  Body_Fixed_Angle/1 -> Demux/1
  Demux/1 -> Trigonometric Function/1, Trigonometric Function1/1
  Trigonometric Function/1 -> [Sin_Phi]
  Trigonometric Function1/1 -> [Cos_Phi]
  Demux/2 -> Trigonometric Function3/1, Trigonometric Function2/1
  Trigonometric Function2/1 -> [Sin_Theta]
  Trigonometric Function3/1 -> [Cos_Theta]
  Trigonometric Function4/1 -> [Sin_Psi]
  Trigonometric Function5/1 -> [Cos_Psi]
  Demux/3 -> Trigonometric Function4/1, Trigonometric Function5/1
  [Cos_Phi] -> Product/1
  [Sin_Theta] -> Product/2
  [Cos_Psi] -> Product/3
  Product/1 -> Sum/1
  [Sin_Phi] -> Product1/1
  [Sin_Psi] -> Product1/2
  Product1/1 -> Sum/2
  Sum/1 -> Product2/2
  Product2/1 -> Gain/1
  [Cos_Phi] -> Product3/1
  [Sin_Theta] -> Product3/2
  [Sin_Psi] -> Product3/3
  Product3/1 -> Sum1/1
  [Sin_Phi] -> Product4/1
  [Cos_Psi] -> Product4/2
  Product4/1 -> Sum1/2
  Sum1/1 -> Product5/2
  Thrust_Force/1 -> Product7/1, Product5/1, Product2/1
  Product5/1 -> Gain1/1
  Gain1/1 -> Mux/2
  [Cos_Phi] -> Product6/1
  [Cos_Theta] -> Product6/2
  Product7/1 -> Gain2/1
  Gain2/1 -> Sum2/2
  Gravity/1 -> Sum2/1
  Product6/1 -> Product7/2
  Gain/1 -> Mux/1
  Sum2/1 -> Mux/3
  Mux/1 -> Integrator1/1
  Integrator1/1 -> Velocity/1

== system QuadSimUnity/Motor and Quadrotor Model/UDP Postion From Unity ==
  Trigger : TriggerPort  PortDimensions=1
  UDP Receive : dspnetwork/UDP Receive  localURL='0.0.0.0'  localPort=3000  remoteURL='127.0.0.1'  remotePort=-1  recvBufferSize=24  dims=12  signalDatatype=uint8  isVarSize=off  showBlockingTime=on  blockingTime=0  sampletime=-1  blockPlatform=HOST
  UDP Stream : Outport
  wires:
  UDP Receive/1 -> UDP Stream/1

== system QuadSimUnity/Motor and Quadrotor Model/Position Control/PID Angle Controller ==
  Angle_Demand : Inport
  Angle_Meas. : Inport  Port=2
  Demux : Demux  Outputs=3
  Demux1 : Demux  Outputs=3
  Mux : Mux  Inputs=3
  PID Controller (2DOF) : simulink/Continuous/PID Controller (2DOF)  Controller=PID  TimeDomain=Continuous-time  SampleTime=-1  IntegratorMethod=Forward Euler  FilterMethod=Forward Euler  Form=Parallel  UseFilter=on  ControllerParametersSource=internal  P=P_angle  I=I_angle  D=D_angle  N=100  b=1  c=1  InitialConditionSource=internal  InitialConditionForIntegrator=0  InitialConditionForFilter=0  ExternalReset=none  LimitOutput=off  UpperSaturationLimit=inf  LowerSaturationLimit=-inf  LinearizeAsGain=on  AntiWindupMode=none  Kb=1  TrackingMode=off  Kt=1  PParamMin=[]  PParamMax=[]  IParamMin=[]  IParamMax=[]  DParamMin=[]  DParamMax=[]  NParamMin=[]  NParamMax=[]  bParamMin=[]  bParamMax=[]  cParamMin=[]  cParamMax=[]  KbParamMin=[]  KbParamMax=[]  KtParamMin=[]  KtParamMax=[]  POutMin=[]  POutMax=[]  IOutMin=[]  IOutMax=[]  DOutMin=[]  DOutMax=[]  NOutMin=[]  NOutMax=[]  bOutMin=[]  bOutMax=[]  cOutMin=[]  cOutMax=[]  KbOutMin=[]  KbOutMax=[]  KtOutMin=[]  KtOutMax=[]  IntegratorOutMin=[]  IntegratorOutMax=[]  FilterOutMin=[]  FilterOutMax=[]  SumOutMin=[]  SumOutMax=[]  Sum1OutMin=[]  Sum1OutMax=[]  Sum2OutMin=[]  Sum2OutMax=[]  Sum3OutMin=[]  Sum3OutMax=[]  SumI1OutMin=[]  SumI1OutMax=[]  SumI2OutMin=[]  SumI2OutMax=[]  SumI3OutMin=[]  SumI3OutMax=[]  SumDOutMin=[]  SumDOutMax=[]  SaturationOutMin=[]  SaturationOutMax=[]  IntegratorContinuousStateAttributes=''  IntegratorStateMustResolveToSignalObject=off  IntegratorRTWStateStorageClass=Auto  FilterContinuousStateAttributes=''  FilterStateMustResolveToSignalObject=off  FilterRTWStateStorageClass=Auto  DifferentiatorICPrevScaledInput=0  DifferentiatorOutMin=[]  DifferentiatorOutMax=[]
  PID Controller (2DOF)1 : simulink/Continuous/PID Controller (2DOF)  Controller=PID  TimeDomain=Continuous-time  SampleTime=-1  IntegratorMethod=Forward Euler  FilterMethod=Forward Euler  Form=Parallel  UseFilter=on  ControllerParametersSource=internal  P=P_angle  I=I_angle  D=D_angle  N=100  b=1  c=1  InitialConditionSource=internal  InitialConditionForIntegrator=0  InitialConditionForFilter=0  ExternalReset=none  LimitOutput=off  UpperSaturationLimit=inf  LowerSaturationLimit=-inf  LinearizeAsGain=on  AntiWindupMode=none  Kb=1  TrackingMode=off  Kt=1  PParamMin=[]  PParamMax=[]  IParamMin=[]  IParamMax=[]  DParamMin=[]  DParamMax=[]  NParamMin=[]  NParamMax=[]  bParamMin=[]  bParamMax=[]  cParamMin=[]  cParamMax=[]  KbParamMin=[]  KbParamMax=[]  KtParamMin=[]  KtParamMax=[]  POutMin=[]  POutMax=[]  IOutMin=[]  IOutMax=[]  DOutMin=[]  DOutMax=[]  NOutMin=[]  NOutMax=[]  bOutMin=[]  bOutMax=[]  cOutMin=[]  cOutMax=[]  KbOutMin=[]  KbOutMax=[]  KtOutMin=[]  KtOutMax=[]  IntegratorOutMin=[]  IntegratorOutMax=[]  FilterOutMin=[]  FilterOutMax=[]  SumOutMin=[]  SumOutMax=[]  Sum1OutMin=[]  Sum1OutMax=[]  Sum2OutMin=[]  Sum2OutMax=[]  Sum3OutMin=[]  Sum3OutMax=[]  SumI1OutMin=[]  SumI1OutMax=[]  SumI2OutMin=[]  SumI2OutMax=[]  SumI3OutMin=[]  SumI3OutMax=[]  SumDOutMin=[]  SumDOutMax=[]  SaturationOutMin=[]  SaturationOutMax=[]  IntegratorContinuousStateAttributes=''  IntegratorStateMustResolveToSignalObject=off  IntegratorRTWStateStorageClass=Auto  FilterContinuousStateAttributes=''  FilterStateMustResolveToSignalObject=off  FilterRTWStateStorageClass=Auto  DifferentiatorICPrevScaledInput=0  DifferentiatorOutMin=[]  DifferentiatorOutMax=[]
  PID Controller (2DOF)2 : simulink/Continuous/PID Controller (2DOF)  Controller=PID  TimeDomain=Continuous-time  SampleTime=-1  IntegratorMethod=Forward Euler  FilterMethod=Forward Euler  Form=Parallel  UseFilter=on  ControllerParametersSource=internal  P=P_angle  I=I_angle  D=D_angle  N=100  b=1  c=1  InitialConditionSource=internal  InitialConditionForIntegrator=0  InitialConditionForFilter=0  ExternalReset=none  LimitOutput=off  UpperSaturationLimit=inf  LowerSaturationLimit=-inf  LinearizeAsGain=on  AntiWindupMode=none  Kb=1  TrackingMode=off  Kt=1  PParamMin=[]  PParamMax=[]  IParamMin=[]  IParamMax=[]  DParamMin=[]  DParamMax=[]  NParamMin=[]  NParamMax=[]  bParamMin=[]  bParamMax=[]  cParamMin=[]  cParamMax=[]  KbParamMin=[]  KbParamMax=[]  KtParamMin=[]  KtParamMax=[]  POutMin=[]  POutMax=[]  IOutMin=[]  IOutMax=[]  DOutMin=[]  DOutMax=[]  NOutMin=[]  NOutMax=[]  bOutMin=[]  bOutMax=[]  cOutMin=[]  cOutMax=[]  KbOutMin=[]  KbOutMax=[]  KtOutMin=[]  KtOutMax=[]  IntegratorOutMin=[]  IntegratorOutMax=[]  FilterOutMin=[]  FilterOutMax=[]  SumOutMin=[]  SumOutMax=[]  Sum1OutMin=[]  Sum1OutMax=[]  Sum2OutMin=[]  Sum2OutMax=[]  Sum3OutMin=[]  Sum3OutMax=[]  SumI1OutMin=[]  SumI1OutMax=[]  SumI2OutMin=[]  SumI2OutMax=[]  SumI3OutMin=[]  SumI3OutMax=[]  SumDOutMin=[]  SumDOutMax=[]  SaturationOutMin=[]  SaturationOutMax=[]  IntegratorContinuousStateAttributes=''  IntegratorStateMustResolveToSignalObject=off  IntegratorRTWStateStorageClass=Auto  FilterContinuousStateAttributes=''  FilterStateMustResolveToSignalObject=off  FilterRTWStateStorageClass=Auto  DifferentiatorICPrevScaledInput=0  DifferentiatorOutMin=[]  DifferentiatorOutMax=[]
  Scope : Scope  NumInputPorts=2
  Sum : Sum  Inputs=|+-
  Angle_Rate_Demand : Outport
  wires:
  Demux1/2 -> PID Controller (2DOF)1/2
  Demux/2 -> PID Controller (2DOF)1/1
  Angle_Meas./1 -> Demux1/1, Sum/2
  Demux1/1 -> PID Controller (2DOF)/2
  Demux/1 -> PID Controller (2DOF)/1
  Demux1/3 -> PID Controller (2DOF)2/2
  Angle_Demand/1 -> Scope/1, Sum/1, Demux/1
  Demux/3 -> PID Controller (2DOF)2/1
  PID Controller (2DOF)/1 -> Mux/1
  PID Controller (2DOF)1/1 -> Mux/2
  PID Controller (2DOF)2/1 -> Mux/3
  Mux/1 -> Angle_Rate_Demand/1
  Sum/1 -> Scope/2

== system QuadSimUnity/Motor and Quadrotor Model/Reference_Postion/UDP Traj Recieve ==
  Trigger : TriggerPort  PortDimensions=1
  Byte Unpack1 : etargetslib/Byte Unpack  dimensions={1,1,1}  datatypes={'double','double','double'}  byteAlign=1
  UDP Receive : dspnetwork/UDP Receive  localURL='0.0.0.0'  localPort=25002  remoteURL='127.0.0.1'  remotePort=-1  recvBufferSize=24  dims=24  signalDatatype=uint8  isVarSize=off  showBlockingTime=on  blockingTime=0  sampletime=-1  blockPlatform=HOST
  xd : Outport
  yd : Outport  Port=2
  zd : Outport  Port=3
  wires:
  UDP Receive/1 -> Byte Unpack1/1
  Byte Unpack1/1 -> xd/1
  Byte Unpack1/2 -> yd/1
  Byte Unpack1/3 -> zd/1

== system QuadSimUnity/Motor and Quadrotor Model/Reference_PostionParamtetrized/Subsystem1 ==
  coefficients : Inport
  s : Inport  Port=2
  polynomial : Product  Multiplication=Matrix(*)  SaturateOnIntegerOverflow=on  OutDataTypeStr=Inherit: Same as first input
  polynomial1 : Product  Multiplication=Matrix(*)  SaturateOnIntegerOverflow=on  OutDataTypeStr=Inherit: Same as first input
  tau vector : Subsystem
  tau vector1 : Subsystem
  pc(s) : Outport
  der : Outport  Port=2
  wires:
  polynomial/1 -> pc(s)/1
  tau vector/1(tau_vector) -> polynomial/2
  tau vector1/1(tau_vector) -> polynomial1/2
  s/1 -> tau vector1/1(tau), tau vector/1(tau)
  coefficients/1 -> polynomial1/1, polynomial/1
  polynomial1/1 -> der/1

== system QuadSimUnity/Motor and Quadrotor Model/Reference_PostionParamtetrized/UDP Traj Recieve ==
  Trigger : TriggerPort  PortDimensions=1
  Byte Unpack1 : etargetslib/Byte Unpack  dimensions={1,1}  datatypes={'int8','int8'}  byteAlign=1
  Data Type Conversion : DataTypeConversion  OutDataTypeStr=double
  Data Type Conversion1 : DataTypeConversion  OutDataTypeStr=double
  UDP Receive : dspnetwork/UDP Receive  localURL='0.0.0.0'  localPort=25002  remoteURL='127.0.0.1'  remotePort=-1  recvBufferSize=2  dims=2  signalDatatype=uint8  isVarSize=off  showBlockingTime=on  blockingTime=0  sampletime=-1  blockPlatform=HOST
  start/stop : Outport
  reset : Outport  Port=2
  wires:
  UDP Receive/1 -> Byte Unpack1/1
  Byte Unpack1/1 -> Data Type Conversion/1
  Byte Unpack1/2 -> Data Type Conversion1/1
  Data Type Conversion/1 -> start/stop/1
  Data Type Conversion1/1 -> reset/1

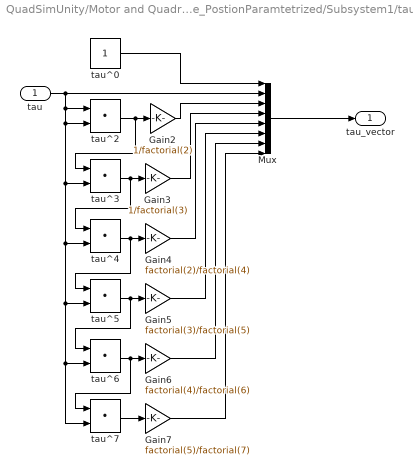
== system QuadSimUnity/Motor and Quadrotor Model/Reference_PostionParamtetrized/Subsystem1/tau vector ==
  tau : Inport
  Gain2 : Gain  Gain=1/factorial(2)  SaturateOnIntegerOverflow=on  OutDataTypeStr=Inherit: Same as input  ParamDataTypeStr=Inherit: Same as input
  Gain3 : Gain  Gain=1/factorial(3)  SaturateOnIntegerOverflow=on  OutDataTypeStr=Inherit: Same as input  ParamDataTypeStr=Inherit: Same as input
  Gain4 : Gain  Gain=factorial(2)/factorial(4)  SaturateOnIntegerOverflow=on  OutDataTypeStr=Inherit: Same as input  ParamDataTypeStr=Inherit: Same as input
  Gain5 : Gain  Gain=factorial(3)/factorial(5)  SaturateOnIntegerOverflow=on  OutDataTypeStr=Inherit: Same as input  ParamDataTypeStr=Inherit: Same as input
  Gain6 : Gain  Gain=factorial(4)/factorial(6)  SaturateOnIntegerOverflow=on  OutDataTypeStr=Inherit: Same as input  ParamDataTypeStr=Inherit: Same as input
  Gain7 : Gain  Gain=factorial(5)/factorial(7)  SaturateOnIntegerOverflow=on  OutDataTypeStr=Inherit: Same as input  ParamDataTypeStr=Inherit: Same as input
  Mux : Mux  Inputs=8
  tau^0 : Constant
  tau^{2..7} (6 alike) : DotProduct  InputSameDT=on  OutDataTypeStr=Inherit: Inherit via internal rule
  tau_vector : Outport
  wires:
  tau^6/1 -> tau^7/1, Gain6/1
  tau^7/1 -> Gain7/1
  Gain7/1 -> Mux/8
  Gain6/1 -> Mux/7
  Gain4/1 -> Mux/5
  Gain5/1 -> Mux/6
  tau^5/1 -> tau^6/1, Gain5/1
  Gain2/1 -> Mux/3
  Gain3/1 -> Mux/4
  tau^4/1 -> tau^5/1, Gain4/1
  tau^2/1 -> Gain2/1, tau^3/1
  tau^0/1 -> Mux/1
  tau^3/1 -> Gain3/1, tau^4/1
  tau/1 -> tau^7/2, tau^6/2, tau^5/2, tau^4/2, tau^3/2, tau^2/2, tau^2/1, Mux/2
  Mux/1 -> tau_vector/1

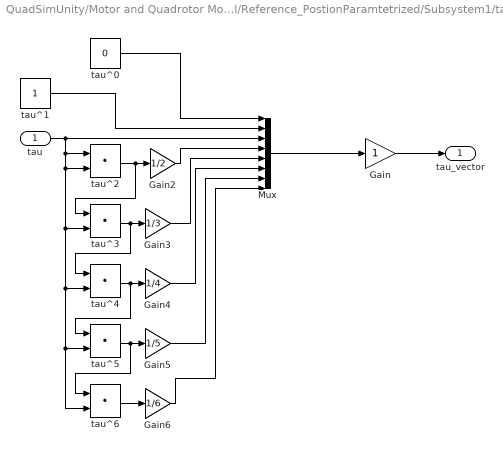
== system QuadSimUnity/Motor and Quadrotor Model/Reference_PostionParamtetrized/Subsystem1/tau vector1 ==
  tau : Inport
  Gain : Gain
  Gain2 : Gain  Gain=1/2  SaturateOnIntegerOverflow=on  OutDataTypeStr=Inherit: Same as input  ParamDataTypeStr=Inherit: Same as input
  Gain3 : Gain  Gain=1/3  SaturateOnIntegerOverflow=on  OutDataTypeStr=Inherit: Same as input  ParamDataTypeStr=Inherit: Same as input
  Gain4 : Gain  Gain=1/4  SaturateOnIntegerOverflow=on  OutDataTypeStr=Inherit: Same as input  ParamDataTypeStr=Inherit: Same as input
  Gain5 : Gain  Gain=1/5  SaturateOnIntegerOverflow=on  OutDataTypeStr=Inherit: Same as input  ParamDataTypeStr=Inherit: Same as input
  Gain6 : Gain  Gain=1/6  SaturateOnIntegerOverflow=on  OutDataTypeStr=Inherit: Same as input  ParamDataTypeStr=Inherit: Same as input
  Mux : Mux  Inputs=8
  tau^0 : Constant  Value=0
  tau^1 : Constant
  tau^{2..6} (5 alike) : DotProduct  InputSameDT=on  OutDataTypeStr=Inherit: Inherit via internal rule
  tau_vector : Outport
  wires:
  Mux/1 -> Gain/1
  tau^0/1 -> Mux/1
  tau/1 -> Mux/3, tau^2/1, tau^2/2, tau^3/2, tau^4/2, tau^5/2, tau^6/2
  tau^3/1 -> tau^4/1, Gain3/1
  tau^2/1 -> tau^3/1, Gain2/1
  tau^4/1 -> Gain4/1, tau^5/1
  Gain3/1 -> Mux/5
  Gain2/1 -> Mux/4
  tau^5/1 -> Gain5/1, tau^6/1
  Gain5/1 -> Mux/7
  Gain4/1 -> Mux/6
  Gain6/1 -> Mux/8
  tau^6/1 -> Gain6/1
  tau^1/1 -> Mux/2
  Gain/1 -> tau_vector/1

== matlab function QuadSimUnity/Motor and Quadrotor Model/Rotation_Dynamic ==
  data: Thrust_real output; u1 output; u3 output; u5 output; u7 output; Moment_xyz_real output; Rtr_Spd_Sqrd input; Moment_Input input; Inertia input; inv_Inertia input; Fail_State input; Param_b_l_d_Jr input; Ang_Vel_RPY input; Ang_Accel_RPY output; Input_Power output; Output_Power output
function [Thrust_real,u1,u3,u5,u7, Moment_xyz_real, Ang_Accel_RPY, Input_Power, Output_Power]  = fcn(Rtr_Spd_Sqrd, Moment_Input, Inertia, inv_Inertia, Fail_State, Param_b_l_d_Jr, Ang_Vel_RPY)
                
b = Param_b_l_d_Jr(1);
l = Param_b_l_d_Jr(2);
d = Param_b_l_d_Jr(3);
Jr = Param_b_l_d_Jr(4);

u1 = Rtr_Spd_Sqrd(1); u2 = Rtr_Spd_Sqrd(2); u3 = Rtr_Spd_Sqrd(3); u4 = Rtr_Spd_Sqrd(4); 
u5 = Rtr_Spd_Sqrd(5); u6 = Rtr_Spd_Sqrd(6); u7 = Rtr_Spd_Sqrd(7); u8 = Rtr_Spd_Sqrd(8); 

Input_Power = sum(Rtr_Spd_Sqrd.*Rtr_Spd_Sqrd);

Output_Power = sum((diag(Fail_State)*Rtr_Spd_Sqrd).*(diag(Fail_State)*Rtr_Spd_Sqrd));

Phi_M = ...
... 
[       0,       0, b*l*u3, b*l*u4,      0,      0, -b*l*u7, -b*l*u8; ...
  -b*l*u1, -b*l*u2,      0,      0, b*l*u5, b*l*u6,       0,       0; ...
    -d*u1,    d*u2,   d*u3,  -d*u4,  -d*u5,   d*u6,    d*u7,   -d*u8];

Phi_T = ...
... 
[ b*u1, b*u2, b*u3, b*u4, b*u5, b*u6, b*u7, b*u8];

Thrust_real = Phi_T * Fail_State;


Rtr_Spd_sum = [sqrt(abs(Rtr_Spd_Sqrd(1)))*sign(Rtr_Spd_Sqrd(1)), ...
             -sqrt(abs(Rtr_Spd_Sqrd(2)))*sign(Rtr_Spd_Sqrd(2)), ...
             sqrt(abs(Rtr_Spd_Sqrd(3)))*sign(Rtr_Spd_Sqrd(3)), ...
             -sqrt(abs(Rtr_Spd_Sqrd(4)))*sign(Rtr_Spd_Sqrd(4)), ...
             sqrt(abs(Rtr_Spd_Sqrd(5)))*sign(Rtr_Spd_Sqrd(5)), ...
             -sqrt(abs(Rtr_Spd_Sqrd(6)))*sign(Rtr_Spd_Sqrd(6)), ...
             sqrt(abs(Rtr_Spd_Sqrd(7)))*sign(Rtr_Spd_Sqrd(7)), ...
             -sqrt(abs(Rtr_Spd_Sqrd(8)))*sign(Rtr_Spd_Sqrd(8))]*Fail_State;

sigma = [-Jr*Ang_Vel_RPY(2)*Rtr_Spd_sum; +Jr*Ang_Vel_RPY(1)*Rtr_Spd_sum; 0];

Moment_xyz_real = Phi_M * Fail_State;

Ang_Accel_RPY = inv_Inertia*(-cross(Ang_Vel_RPY,(Inertia*Ang_Vel_RPY)) + sigma + Moment_xyz_real+ Moment_Input);
